simulink model "Model_Mk2"  (R2022b)
settings: Solver=VariableStepAuto  StartTime=0.0  StopTime=5  FixedStep=1e-6  EnableMultiTasking=on
model workspace: external: MATLAB File C:\Users\anigo\OneDrive\Documents\GitHub\Modeling-and-control\getParams.m (data not in the file)
values from neighbouring files (symbols this model uses):
  g = 9.81    [getParams.m]    (also in get_segment_traj.m = consts(3))
  l = raw(4, 2)    [getParams.m]    (also in get_segment_traj.m = consts(2))
  m = 4    [Moi_Tensor.m]    (also in getParams.m = raw(5, 2); get_segment_traj.m = consts(1); noise_calculation.m = unique(m))
  MOI = raw(1:3, 2:4)    [getParams.m]
  x1 = [10; 5; 5; 0; 0; 0; q1; 0; 0; 0]    [getParams.m]    (also in get_trajectory.m = x(1))
undefined symbols (not defined in the file or in its folder): Kset, t_set, tSegs, u_set, x_set
libraries: sharedtransform x2, vrlib x2
settings Model: Creator=davis  LastModifiedBy=anigo
settings SolverCC: ZeroCrossAlgorithm=Adaptive  PositivePriorityOrder=on
settings OptimizationCC: DefaultParameterBehavior=Inlined  EnhancedBackFolding=on  PassReuseOutputArgsAs=Individual arguments  ZeroExternalMemoryAtStartup=off  ZeroInternalMemoryAtStartup=off  MaxStackSize=64  OptimizeBlockOrder=speed  DifferentSizesBufferReuse=on  OptimizationCustomize=off  EfficientTunableParamExpr=on
settings DebuggingCC: IgnoredZcDiagnostic=none  ParameterTunabilityLossMsg=error  UnconnectedInputMsg=warning  UnconnectedOutputMsg=warning  UnconnectedLineMsg=warning
settings HardwareCC: ProdBitPerPointer=32  ProdBitPerSizeT=32  ProdBitPerPtrDiffT=32  ProdLargestAtomicInteger=Long  ProdLargestAtomicFloat=Double  ProdWordSize=32  ProdHWDeviceType=ARM Compatible->ARM Cortex-M  HardwareBoardFeatureSet=SoCBlockset
settings ModelReferenceCC: UpdateModelReferenceTargets=Force  EnableRefExpFcnMdlSchedulingChecks=on  ModelReferenceNumInstancesAllowed=Single
settings SFSimCC: MATLABDynamicMemAlloc=off
settings RTWCC: Description=Embedded Coder  SystemTargetFile=ert.tlc  TemplateMakefile=ert_default_tmf  DLArmComputeVersion=19.05
settings CodeAppCC: ForceParamTrailComments=on  IgnoreCustomStorageClasses=off  OperatorAnnotations=on  SimulinkDataObjDesc=on  SFDataObjDesc=on  InsertBlockDesc=on
settings ERTTargetCC: ERTCustomFileTemplate=example_file_process.tlc

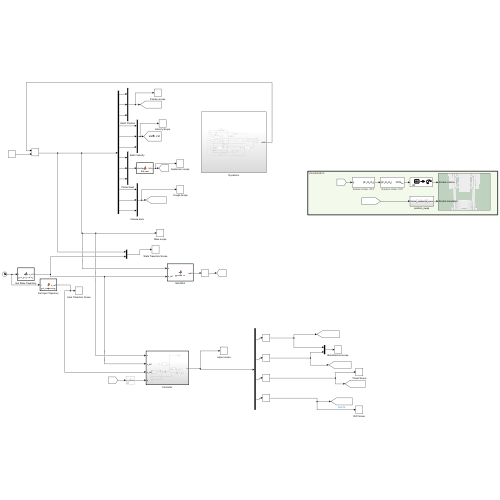
[thumbnail: Simulink's stored preview of the top-level diagram]
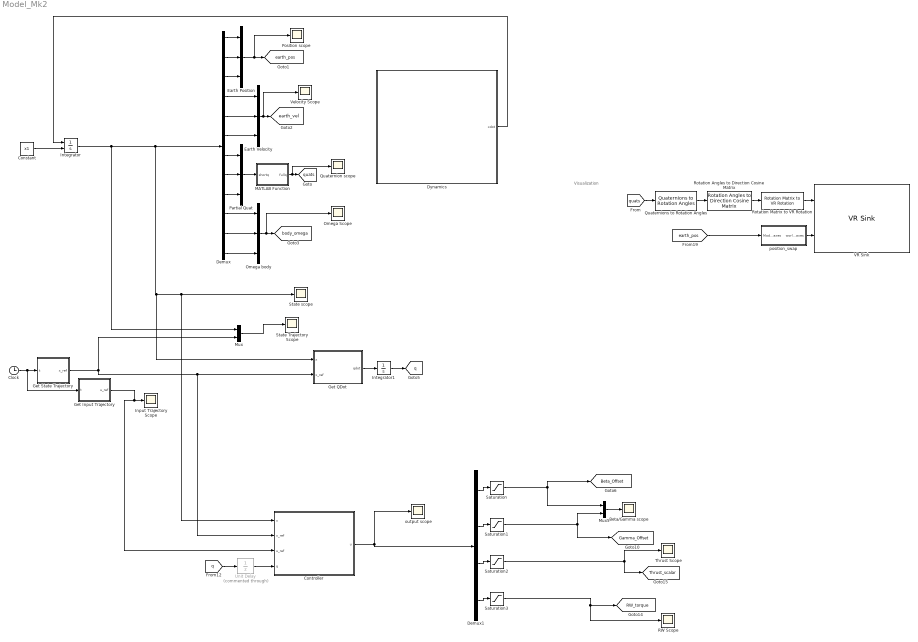
== system Model_Mk2 ==
  note: Visualization
  Beta/Gamma scope : Scope
  Clock : Clock
  Constant : Constant  Value=x1
  Controller : Subsystem  TreatAsAtomicUnit=on
      settings: MinAlgLoopOccurrences=on
      settings: LibrarySourceBlock=|
      | hdlsllib/Ports &
      | Subsystems/Triggered
      | Subsystem
  Demux : Demux  Outputs=12
  Demux1 : Demux
  Dynamics : Subsystem
  Earth Position : Mux  Inputs=3
  Earth Velocity : Mux  Inputs=3
  Get Input Trajectory : MATLAB Function  TreatAsAtomicUnit=on
  Get QDot : MATLAB Function  TreatAsAtomicUnit=on
  Get State Trajectory : MATLAB Function  TreatAsAtomicUnit=on
  Input Trajectory Scope : Scope
  Integrator : Integrator  InitialConditionSource=external
  Integrator1 : Integrator
  MATLAB Function : MATLAB Function  TreatAsAtomicUnit=on
  Mux : Mux  Inputs=2
  Mux5 : Mux  Inputs=2
  Omega Scope : Scope
  Omega body : Mux  Inputs=3
  Partial Quat : Mux  Inputs=3
  Position scope : Scope
  Quaternion scope : Scope
  Quaternions to Rotation Angles : sharedtransform/Quaternions to Rotation Angles  rotationOrder=ZYX  aMode=aMode
  RW Scope : Scope
  Rotation Angles to Direction Cosine Matrix : sharedtransform/Rotation Angles to Direction Cosine Matrix  rotationOrder=ZYX  aMode=aMode
  Rotation Matrix to VR Rotation : vrlib/Utilities/Rotation Matrix to VR Rotation  maxzero=1e-12
  Saturation : Saturate  UpperLimit=pi/12  LowerLimit=-pi/12  LinearizeAsGain=off
  Saturation1 : Saturate  UpperLimit=pi/12  LowerLimit=-pi/12  LinearizeAsGain=off
  Saturation2 : Saturate  UpperLimit=400  LowerLimit=0  LinearizeAsGain=off  ZeroCross=off
  Saturation3 : Saturate  UpperLimit=2  LowerLimit=-2  LinearizeAsGain=off
  State Trajectory Scope : Scope
  State scope : Scope
  Thrust Scope : Scope
  Unit Delay : UnitDelay  Commented=through  SampleTime=-1  HasFrameUpgradeWarning=on
  VR Sink : vrlib/VR Sink  InstantiateOnLoad=on  SampleTime=0.1  ViewEnable=on  RemoteChange=off  RemoteView=off  FieldsWritten=Rocket.rotation.4.1.1.double#Rocket.translation.3.1.1.double  WorldFileName=world.x3d  AutoView=off  VideoDimensions=[]  AllowVariableSize=off
  Velocity Scope : Scope
  output scope : Scope
  position_swap : Subsystem
  tag scope: Beta_Offset=global, Gamma_Offset=global, RW_torque=global, Thrust_scalar=global, body_omega=global, earth_pos=global, earth_vel=global, q=global, quats=global
  wires:
  Rotation Matrix to VR Rotation/1 -> VR Sink/1
  position_swap/1(world_axes) -> VR Sink/2
  Saturation/1 -> Mux5/1, [Beta_Offset]
  Saturation1/1 -> [Gamma_Offset], Mux5/2
  Saturation3/1 -> RW Scope/1, [RW_torque]
  Clock/1 -> Get Input Trajectory/1(t), Get State Trajectory/1(t)
  Demux1/1 -> Saturation/1
  Mux5/1 -> Beta/Gamma scope/1
  Saturation2/1 -> [Thrust_scalar], Thrust Scope/1
  Demux1/4 -> Saturation3/1
  Demux1/2 -> Saturation1/1
  Demux1/3 -> Saturation2/1
  Controller/1(u) -> Demux1/1, output scope/1
  Unit Delay/1 -> Controller/4(q)
  [q] -> Unit Delay/1
  Get Input Trajectory/1(u_ref) -> Controller/3(u_ref), Input Trajectory Scope/1
  Get State Trajectory/1(x_ref) -> Controller/2(x_ref), Get QDot/2(x_ref), Mux/2
  Constant/1 -> Integrator/2
  Integrator/1 -> Mux/1, Get QDot/1(x), Controller/1(x), State scope/1, Demux/1
  Demux/3 -> Earth Position/3
  Demux/2 -> Earth Position/2
  Demux/4 -> Earth Velocity/1
  Demux/5 -> Earth Velocity/2
  Demux/6 -> Earth Velocity/3
  Demux/7 -> Partial Quat/1
  Demux/8 -> Partial Quat/2
  Demux/9 -> Partial Quat/3
  Demux/10 -> Omega body/1
  Demux/11 -> Omega body/2
  Demux/12 -> Omega body/3
  Partial Quat/1 -> MATLAB Function/1(shortq)
  Earth Position/1 -> Position scope/1, [earth_pos]
  Dynamics/1(xdot) -> Integrator/1
  Demux/1 -> Earth Position/1
  Omega body/1 -> Omega Scope/1, [body_omega]
  Earth Velocity/1 -> Velocity Scope/1, [earth_vel]
  MATLAB Function/1(fullq) -> Quaternion scope/1, [quats]
  Rotation Angles to Direction Cosine Matrix/1 -> Rotation Matrix to VR Rotation/1
  Quaternions to Rotation Angles/1 -> Rotation Angles to Direction Cosine Matrix/1
  [quats] -> Quaternions to Rotation Angles/1
  [earth_pos] -> position_swap/1(Model_axes)
  Get QDot/1(qdot) -> Integrator1/1
  Integrator1/1 -> [q]
  Mux/1 -> State Trajectory Scope/1

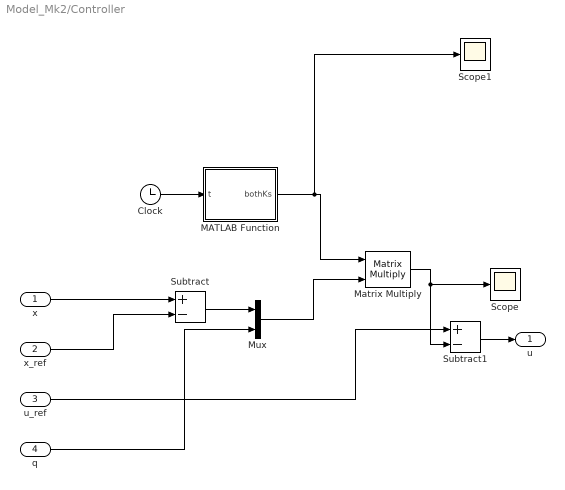
== system Model_Mk2/Controller ==
  x : Inport
  x_ref : Inport  Port=2
  u_ref : Inport  Port=3
  q : Inport  Port=4
  Clock : Clock
  MATLAB Function : MATLAB Function  TreatAsAtomicUnit=on
  Matrix Multiply : Product  Multiplication=Matrix(*)
  Mux : Mux  Inputs=2
  Scope : Scope
  Scope1 : Scope
  Subtract : Sum  Inputs=+-
  Subtract1 : Sum  Inputs=+-
  u : Outport
  wires:
  x/1 -> Subtract/1
  x_ref/1 -> Subtract/2
  Subtract/1 -> Mux/1
  q/1 -> Mux/2
  Clock/1 -> MATLAB Function/1(t)
  MATLAB Function/1(bothKs) -> Scope1/1, Matrix Multiply/1
  Mux/1 -> Matrix Multiply/2
  u_ref/1 -> Subtract1/1
  Matrix Multiply/1 -> Scope/1, Subtract1/2
  Subtract1/1 -> u/1

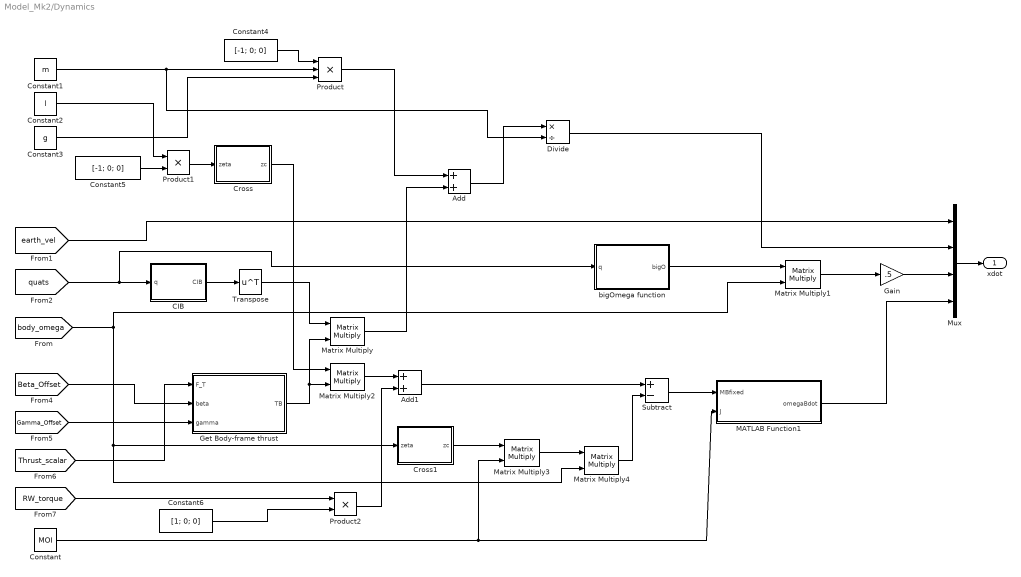
== system Model_Mk2/Dynamics ==
  Add : Sum
  Add1 : Sum
  CIB : MATLAB Function  TreatAsAtomicUnit=on
  Constant : Constant  Value=MOI
  Constant1 : Constant  Value=m
  Constant2 : Constant  Value=l
  Constant3 : Constant  Value=g
  Constant4 : Constant  Value=[-1; 0; 0]
  Constant5 : Constant  Value=[-1; 0; 0]
  Constant6 : Constant  Value=[1; 0; 0]
  Cross : MATLAB Function  TreatAsAtomicUnit=on
  Cross1 : MATLAB Function  TreatAsAtomicUnit=on
  Divide : Product  Inputs=*/
  Gain : Gain  Gain=.5
  Get Body-frame thrust : MATLAB Function  TreatAsAtomicUnit=on
  MATLAB Function1 : MATLAB Function  TreatAsAtomicUnit=on
  Matrix Multiply{,1..4} (5 alike) : Product  Multiplication=Matrix(*)
  Mux : Mux
  Product : Product  Inputs=3
  Product1 : Product
  Product2 : Product
  Subtract : Sum  Inputs=+-
  Transpose : Math  Operator=transpose
  bigOmega function : MATLAB Function  TreatAsAtomicUnit=on
  xdot : Outport
  wires:
  [quats] -> bigOmega function/1(q), CIB/1(q)
  [Thrust_scalar] -> Get Body-frame thrust/1(F_T)
  [Beta_Offset] -> Get Body-frame thrust/2(beta)
  [Gamma_Offset] -> Get Body-frame thrust/3(gamma)
  CIB/1(CIB) -> Transpose/1
  Transpose/1 -> Matrix Multiply/1
  Get Body-frame thrust/1(TB) -> Matrix Multiply/2, Matrix Multiply2/2
  Constant4/1 -> Product/1
  Constant1/1 -> Divide/2, Product/2
  Constant3/1 -> Product/3
  Product/1 -> Add/1
  Matrix Multiply/1 -> Add/2
  Add/1 -> Divide/1
  [body_omega] -> Matrix Multiply4/2, Cross1/1(zeta), Matrix Multiply1/2
  bigOmega function/1(bigO) -> Matrix Multiply1/1
  Matrix Multiply1/1 -> Gain/1
  Constant5/1 -> Product1/2
  Constant2/1 -> Product1/1
  Product1/1 -> Cross/1(zeta)
  Cross/1(zc) -> Matrix Multiply2/1
  Constant6/1 -> Product2/2
  [RW_torque] -> Product2/1
  Matrix Multiply2/1 -> Add1/1
  Product2/1 -> Add1/2
  Add1/1 -> Subtract/1
  Cross1/1(zc) -> Matrix Multiply3/1
  Constant/1 -> Matrix Multiply3/2, MATLAB Function1/2(J)
  Matrix Multiply3/1 -> Matrix Multiply4/1
  Matrix Multiply4/1 -> Subtract/2
  Subtract/1 -> MATLAB Function1/1(MBfixed)
  Mux/1 -> xdot/1
  [earth_vel] -> Mux/1
  Divide/1 -> Mux/2
  Gain/1 -> Mux/3
  MATLAB Function1/1(omegaBdot) -> Mux/4

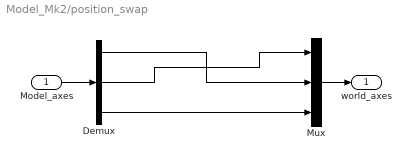
== system Model_Mk2/position_swap ==
  Model_axes : Inport
  Demux : Demux  Outputs=3
  Mux : Mux  Inputs=3
  world_axes : Outport
  wires:
  Demux/3 -> Mux/3
  Demux/2 -> Mux/1
  Mux/1 -> world_axes/1
  Demux/1 -> Mux/2
  Model_axes/1 -> Demux/1

== matlab function Model_Mk2/Get QDot ==
  data: x input; qdot output; x_ref input
function qdot = getQDot(x, x_ref)
C = [eye(3), zeros(3, length(x) - 3)];
qdot = C*x - x_ref(1:3);

== matlab function Model_Mk2/Get State Trajectory ==
  data: t input; x_ref output; x_set parameter; t_set parameter
function x_ref = get_trajectory(t, x_set, t_set)
    x_ref = zeros(size(x_set, 1), 1);
    for i = 1:size(x_ref, 1)
        x_ref(i) = interp1(t_set, x_set(i, :), t);
    end
end

== matlab function Model_Mk2/Controller/MATLAB Function ==
  data: t input; bothKs output; Kset parameter; tSegs parameter
function bothKs = fcn(t, Kset, tSegs)
currentIndex = -1;
for i = 1:length(tSegs)
    if t < tSegs(i)
        currentIndex = i-1;
        break;
    end
end

bothKs = Kset(:, :, currentIndex);

== matlab function Model_Mk2/Get Input Trajectory ==
  data: t input; u_ref output; u_set parameter; t_set parameter
function u_ref = get_trajectory(t, u_set, t_set)
    u_ref = zeros(size(u_set, 1), 1);
    for i = 1:size(u_set, 1)
        u_ref(i) = interp1(t_set, u_set(i, :), t);
    end
end

== matlab function Model_Mk2/Dynamics/CIB ==
  data: q input; CIB output
function CIB = quatRot(q)
    q0 = q(1);
    q1 = q(2);
    q2 = q(3);
    q3 = q(4);
    CIB = [1-2*(q2^2 + q3^2), 2*(q1*q2 + q0*q3), 2*(q1*q3 - q0*q2);
        2*(q1*q2 - q0*q3), 1-2*(q1^2 + q3^2), 2*(q2*q3 + q0*q1);
        2*(q1*q3 + q0*q2), 2*(q2*q3 - q0*q1), 1-2*(q1^2 + q2^2)];
end

== matlab function Model_Mk2/MATLAB Function ==
  data: shortq input size=3; fullq output size=[4 1]
function fullq = fillQuat(shortq)
    q0 = sqrt(1 - (shortq(1)^2) - (shortq(2)^2) - (shortq(3)^2));
    fullq = [q0; shortq];
end

== matlab function Model_Mk2/Dynamics/Get Body-frame thrust ==
  data: F_T input; TB output; beta input; gamma input
function TB = body_thrust(F_T, beta, gamma)
TB = F_T * [cos(beta)*cos(gamma); cos(beta)*sin(gamma); -sin(beta)];
end

== matlab function Model_Mk2/Dynamics/bigOmega function ==
  data: q input size=[4 1]; bigO output
function bigO = bigOmega(q)
    bigO = [q(1) -q(4) q(3); q(4) q(1) -q(2); -q(3) q(2) q(1)];
end

== matlab function Model_Mk2/Dynamics/Cross ==
  data: zeta input; zc output
function zc = zetaCross(zeta)
    zc = [0 -zeta(3) zeta(2); zeta(3) 0 -zeta(1); -zeta(2) zeta(1) 0];
end

== matlab function Model_Mk2/Dynamics/Cross1 ==
  data: zeta input size=[3 1]; zc output
function zc = zetaCross(zeta)
    zc = [0 -zeta(3) zeta(2); zeta(3) 0 -zeta(1); -zeta(2) zeta(1) 0];
end

== matlab function Model_Mk2/Dynamics/MATLAB Function1 ==
  data: MBfixed input; omegaBdot output; J input
function omegaBdot = netAngAcc(MBfixed, J)
    omegaBdot = J \ MBfixed;
end
